simulink model "pull_rod"  (R2019b)
settings: Solver=VariableStepAuto  StartTime=0.0  StopTime=60  RelTol=1e-3
values from neighbouring files (symbols this model uses):
  b = 2000    [Aarm_Disp.m]    (also in Car_Parameters.m; PRdyn.m = 700)
  b_base = wheelbase - a    (= 0.7624)    [Aarm_Disp.m]
  bb = 2000    [Aarm_Disp.m]
  cg_height = .3987    (= 0.3987)    [Aarm_Disp.m]
  gravity = 9.81    [Aarm_Disp.m]
  H = cg_height - e    [Aarm_Disp.m]
  Kf = sf^2*ks/1375    (= 7.06492814545)    [Aarm_Disp.m]
  Kr = sr^2*ksb/1375    (= 8.08978829446)    [Aarm_Disp.m]
  ks = 52538    [Aarm_Disp.m]    (also in Car_Parameters.m = 43781.7; PRdyn.m = 43781.7)
  ksb = 61294.38    [Aarm_Disp.m]
  kt = 600    [Aarm_Disp.m]    (also in Car_Parameters.m = 81.64; PRdyn.m = 81.64)
  ktb = 600    [Aarm_Disp.m]
  l3 = .0807    (= 0.0807)    [Aarm_Disp.m]    (also in Car_Parameters.m = 0.1016; PRdyn.m = 0.1016)
  l3b = .0774    (= 0.0774)    [Aarm_Disp.m]
  l4 = .0358    (= 0.0358)    [Aarm_Disp.m]    (also in Car_Parameters.m = 0.0508; PRdyn.m = 0.0508)
  l4b = .0628    (= 0.0628)    [Aarm_Disp.m]
  mc = 63.5    [Aarm_Disp.m]    (also in Car_Parameters.m = 43; PRdyn.m = 43)
  mcb = 72.57    [Aarm_Disp.m]
  mt = 6.649    [Aarm_Disp.m]    (also in Car_Parameters.m = 12.59; PRdyn.m = 12.59)
  mtb = 11.19    [Aarm_Disp.m]
  percentage_antidive = .32    (= 0.32)    [Aarm_Disp.m]
  rch_front = 0.058    [Aarm_Disp.m]
  rch_rear = .0887    (= 0.0887)    [Aarm_Disp.m]
  total_vehicle_mass = 272.16    [Aarm_Disp.m]
  track_front = 1.168    [Aarm_Disp.m]
  track_rear = 1.143    [Aarm_Disp.m]
  wheelbase = 1.626    [Aarm_Disp.m]
undefined symbols (not defined in the file or in its folder): sigbuilder_block
settings Model: Creator=masonpesson  LastModifiedBy=masonpesson

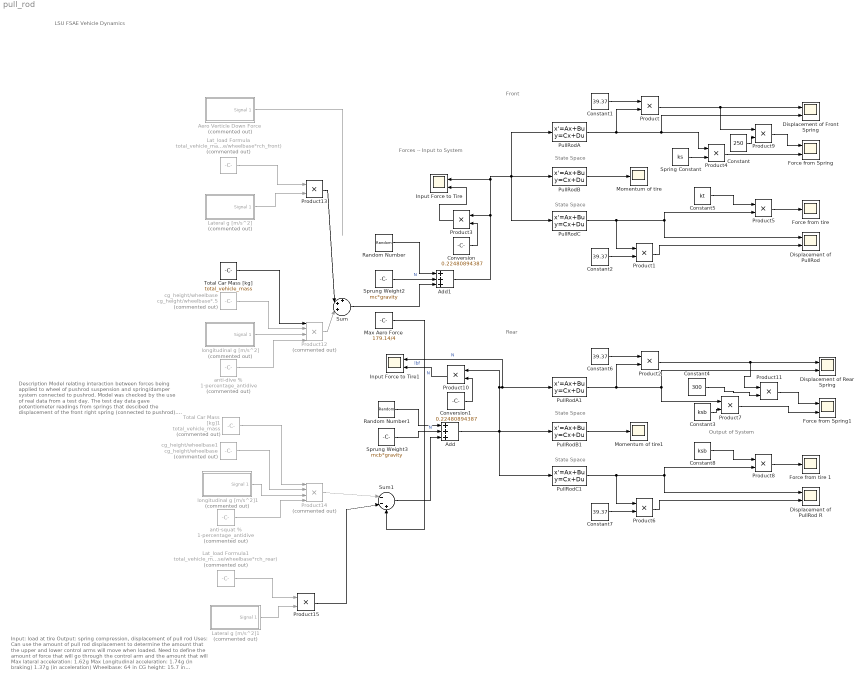
== system pull_rod ==
  note: Input: load at tire
      | Output: spring compression, displacement of pull rod
      |
      | Uses: Can use the amount of pull rod displacement to
      | determine the amount that the upper and lower control
      | arms will move when loaded.
      |
      | Need to define the amount of force that will go through
      | the control arm and the amount that will
      |
      | Max lateral acceleration: 1.62g
      | Max Longitudinal acceleration: 1.74g (in braking)
      | 								  1.37g (in acceleration)
      |
      | Wheelbase: 64 in
      | CG height: 15.7 in
      |
      | Estimated 8 % anti dive:
  note: Rear
  note: State Space
  note: Forces -- Input to System
  note: LSU FSAE Vehicle Dynamics
  note: Description
      |
      | Model relating interaction between forces being applied to wheel of pushrod suspension and spring/damper system connected to pushrod. Model was checked by the use of real data from a test day. The test day data gave potentiometer readings from springs that descibed the displacement of the front right spring (connected to pushrod). This displacement data was then used to calculate the force applied to springs. Those forces were used as an input to this model. The output the model gave was nearly identical to the actual displacment of the springs from the potentiometer data. Note that they were not exactly identical due to the model not having exact measurments but used guessed parameters. More accuate parameters will be pursued.
      |
      | Parameters
      |
      | mt %kg mass of tire --- inertia effects
      | mc %kg coner weight on tire --- force
      | kt %N/m spring in tire
      | ks %N/m spring in actual spring
      | b %Ns/m damping friction
      | l3 %m length to pull rod
      | l4 %m length to spring and damper
      | g %m/s^2 gravityGPS_Altitudem
      |
      | Found Under: Car_Parameters.m
  note: State Space
  note: State Space
  note: State Space
  note: Output of System
  note: Front
  Add : Sum  Inputs=+++
  Add1 : Sum  Inputs=+++
  Aero Verticle Down Force : Subsystem  Tag=STV Subsys  Commented=on  LoadFcn=sigbuilder_block('load');  StartFcn=sigbuilder_block('start');  StopFcn=sigbuilder_block('stop');  ClipboardFcn=sigbuilder_block('clipboard');  mask(Sigbuilder block){tuvar=[0:10]}
      mask help: Simulink:masks:SigbuilderBlock_MD
      mask init:
      | if ~strcmp(get_param(bdroot(gcbh),'SimulationStatus'),'stopped') tuvar = sigbuilder_block('maskInit'); end
      settings: CopyFcn=sigbuilder_block('copy');  DeleteFcn=sigbuilder_block('delete');  ModelCloseFcn=sigbuilder_block('modelClose');  PreSaveFcn=sigbuilder_block('preSave');  PauseFcn=sigbuilder_block('pause');  ContinueFcn=sigbuilder_block('continue');  NameChangeFcn=sigbuilder_block('namechange');  OpenFcn=sigbuilder_block('open',[437.6 199.2 550.4 400 ]);  CloseFcn=sigbuilder_block('close');
      mask Display: plot(0, 0, 100, 100,[2, 2, 32, 32, 2], [68, 8, 8, 68, 68],[32, 2], [38, 38], [32, 19, 2],[53, 60, 44], [32, 17, 17, 2],[16, 16, 31, 31]);txt = getActiveGroup(gcbh);text(2, 100, txt,'verticalAlignment', 'top');
  Constant : Constant  Value=250
  Constant{1..2,6..7} (4 alike) : Constant  Value=39.37
  Constant3 : Constant  Value=ksb
  Constant4 : Constant  Value=300
  Constant5 : Constant  Value=kt
  Constant8 : Constant  Value=ksb
  Conversion : Constant  Value=0.22480894387
  Conversion1 : Constant  Value=0.22480894387
  "Displacement of Front Spring " : Scope  NumInputPorts=2
  Displacement of PullRod : Scope  NumInputPorts=2
  Displacement of PullRod R : Scope  NumInputPorts=2
  Displacement of Rear Spring : Scope  NumInputPorts=2
  Force from Spring : Scope  NumInputPorts=2
  Force from Spring1 : Scope  NumInputPorts=2
  "Force from tire " : Scope
  Force from tire 1 : Scope
  Input Force to Tire : Scope  NumInputPorts=2
  Input Force to Tire1 : Scope  NumInputPorts=2
  Lat_load Formula : Constant  Commented=on  Value=total_vehicle_mass/track_front*((H*Kf/(Kf+Kr)) + b_base/wheelbase*rch_front)
  Lat_load Formula1 : Constant  Commented=on  Value=total_vehicle_mass/track_rear*((H*Kr/(Kr+Kf)) + b_base/wheelbase*rch_rear)
  Lateral g [m/s^2] : Subsystem  Tag=STV Subsys  Commented=on  LoadFcn=sigbuilder_block('load');  StartFcn=sigbuilder_block('start');  StopFcn=sigbuilder_block('stop');  ClipboardFcn=sigbuilder_block('clipboard');  mask(Sigbuilder block){tuvar=[0:10]}
      mask help: Simulink:masks:SigbuilderBlock_MD
      mask init:
      | if ~strcmp(get_param(bdroot(gcbh),'SimulationStatus'),'stopped') tuvar = sigbuilder_block('maskInit'); end
      settings: CopyFcn=sigbuilder_block('copy');  DeleteFcn=sigbuilder_block('delete');  ModelCloseFcn=sigbuilder_block('modelClose');  PreSaveFcn=sigbuilder_block('preSave');  PauseFcn=sigbuilder_block('pause');  ContinueFcn=sigbuilder_block('continue');  NameChangeFcn=sigbuilder_block('namechange');  OpenFcn=sigbuilder_block('open',[437.6 199.2 550.4 400 ]);  CloseFcn=sigbuilder_block('close');
      mask Display: plot(0, 0, 100, 100,[2, 2, 32, 32, 2], [68, 8, 8, 68, 68],[32, 2], [38, 38], [32, 19, 2],[53, 60, 44], [32, 17, 17, 2],[16, 16, 31, 31]);txt = getActiveGroup(gcbh);text(2, 100, txt,'verticalAlignment', 'top');
  Lateral g [m/s^2]1 : Subsystem  Tag=STV Subsys  Commented=on  LoadFcn=sigbuilder_block('load');  StartFcn=sigbuilder_block('start');  StopFcn=sigbuilder_block('stop');  ClipboardFcn=sigbuilder_block('clipboard');  mask(Sigbuilder block){tuvar=[0:10]}
      mask help: Simulink:masks:SigbuilderBlock_MD
      mask init:
      | if ~strcmp(get_param(bdroot(gcbh),'SimulationStatus'),'stopped') tuvar = sigbuilder_block('maskInit'); end
      settings: CopyFcn=sigbuilder_block('copy');  DeleteFcn=sigbuilder_block('delete');  ModelCloseFcn=sigbuilder_block('modelClose');  PreSaveFcn=sigbuilder_block('preSave');  PauseFcn=sigbuilder_block('pause');  ContinueFcn=sigbuilder_block('continue');  NameChangeFcn=sigbuilder_block('namechange');  OpenFcn=sigbuilder_block('open',[437.6 199.2 550.4 400 ]);  CloseFcn=sigbuilder_block('close');
      mask Display: plot(0, 0, 100, 100,[2, 2, 32, 32, 2], [68, 8, 8, 68, 68],[32, 2], [38, 38], [32, 19, 2],[53, 60, 44], [32, 17, 17, 2],[16, 16, 31, 31]);txt = getActiveGroup(gcbh);text(2, 100, txt,'verticalAlignment', 'top');
  Max Aero Force : Constant  Value=179.14/4
  Momentum of tire : Scope
  Momentum of tire1 : Scope
  Product{,1..11,13,15} (14 alike) : Product
  Product12 : Product  Commented=on  Inputs=4
  Product14 : Product  Commented=on  Inputs=4
  PullRodA : StateSpace  A=[0 l3/(l4*mt) 0; -l3/l4*ks -(l3/l4)^2*b/mt -kt; 0 1/mt 0]  B=[0; 1; 0]  C=[1 0 0]  D=0  InitialCondition=0
  PullRodA1 : StateSpace  A=[0 l3b/(l4b*mtb) 0; -l3b/l4b*ksb -(l3b/l4b)^2*bb/mtb -ktb; 0 1/mtb 0]  B=[0; 1; 0]  C=[1 0 0]  D=0  InitialCondition=0
  PullRodB : StateSpace  A=[0 l3/(l4*mt) 0; -l3/l4*ks -(l3/l4)^2*b/mt -kt; 0 1/mt 0]  B=[0; 1; 0]  C=[0 1 0]  D=0  InitialCondition=0
  PullRodB1 : StateSpace  A=[0 l3b/(l4b*mtb) 0; -l3b/l4b*ksb -(l3b/l4b)^2*bb/mtb -ktb; 0 1/mtb 0]  B=[0; 1; 0]  C=[0 1 0]  D=0  InitialCondition=0
  PullRodC : StateSpace  A=[0 l3/(l4*mt) 0; -l3/l4*ks -(l3/l4)^2*b/mt -kt; 0 1/mt 0]  B=[0; 1; 0]  C=[0 0 1]  D=0  InitialCondition=0
  PullRodC1 : StateSpace  A=[0 l3b/(l4b*mtb) 0; -l3b/l4b*ksb -(l3b/l4b)^2*bb/mtb -ktb; 0 1/mtb 0]  B=[0; 1; 0]  C=[0 0 1]  D=0  InitialCondition=0
  Random Number : RandomNumber  Variance=200  SampleTime=.7
  Random Number1 : RandomNumber  Variance=200  SampleTime=.7
  Spring Constant : Constant  Value=ks
  Sprung Weight2 : Constant  Value=mc*gravity
  Sprung Weight3 : Constant  Value=mcb*gravity
  Sum : Sum  Inputs=+++|
  Sum1 : Sum  Inputs=|--+
  Total Car Mass [kg] : Constant  Value=total_vehicle_mass
  Total Car Mass [kg]1 : Constant  Commented=on  Value=total_vehicle_mass
  anti-dive % : Constant  Commented=on  Value=1-percentage_antidive
  anti-squat % : Constant  Commented=on  Value=1-percentage_antidive
  cg_height/wheelbase : Constant  Commented=on  Value=cg_height/wheelbase*.5
  cg_height/wheelbase1 : Constant  Commented=on  Value=cg_height/wheelbase
  longitudinal g [m/s^2] : Subsystem  Tag=STV Subsys  Commented=on  LoadFcn=sigbuilder_block('load');  StartFcn=sigbuilder_block('start');  StopFcn=sigbuilder_block('stop');  ClipboardFcn=sigbuilder_block('clipboard');  mask(Sigbuilder block){tuvar=[0:10]}
      mask help: Simulink:masks:SigbuilderBlock_MD
      mask init:
      | if ~strcmp(get_param(bdroot(gcbh),'SimulationStatus'),'stopped') tuvar = sigbuilder_block('maskInit'); end
      settings: CopyFcn=sigbuilder_block('copy');  DeleteFcn=sigbuilder_block('delete');  ModelCloseFcn=sigbuilder_block('modelClose');  PreSaveFcn=sigbuilder_block('preSave');  PauseFcn=sigbuilder_block('pause');  ContinueFcn=sigbuilder_block('continue');  NameChangeFcn=sigbuilder_block('namechange');  OpenFcn=sigbuilder_block('open',[437.6 199.2 550.4 400 ]);  CloseFcn=sigbuilder_block('close');
      mask Display: plot(0, 0, 100, 100,[2, 2, 32, 32, 2], [68, 8, 8, 68, 68],[32, 2], [38, 38], [32, 19, 2],[53, 60, 44], [32, 17, 17, 2],[16, 16, 31, 31]);txt = getActiveGroup(gcbh);text(2, 100, txt,'verticalAlignment', 'top');
  longitudinal g [m/s^2]1 : Subsystem  Tag=STV Subsys  Commented=on  LoadFcn=sigbuilder_block('load');  StartFcn=sigbuilder_block('start');  StopFcn=sigbuilder_block('stop');  ClipboardFcn=sigbuilder_block('clipboard');  mask(Sigbuilder block){tuvar=[0:10]}
      mask help: Simulink:masks:SigbuilderBlock_MD
      mask init:
      | if ~strcmp(get_param(bdroot(gcbh),'SimulationStatus'),'stopped') tuvar = sigbuilder_block('maskInit'); end
      settings: CopyFcn=sigbuilder_block('copy');  DeleteFcn=sigbuilder_block('delete');  ModelCloseFcn=sigbuilder_block('modelClose');  PreSaveFcn=sigbuilder_block('preSave');  PauseFcn=sigbuilder_block('pause');  ContinueFcn=sigbuilder_block('continue');  NameChangeFcn=sigbuilder_block('namechange');  OpenFcn=sigbuilder_block('open',[437.6 199.2 550.4 400 ]);  CloseFcn=sigbuilder_block('close');
      mask Display: plot(0, 0, 100, 100,[2, 2, 32, 32, 2], [68, 8, 8, 68, 68],[32, 2], [38, 38], [32, 19, 2],[53, 60, 44], [32, 17, 17, 2],[16, 16, 31, 31]);txt = getActiveGroup(gcbh);text(2, 100, txt,'verticalAlignment', 'top');
  wires:
  PullRodA/1 -> Product/2, Product4/1, "Displacement of Front Spring "/2
  PullRodB/1 -> Momentum of tire/1
  Constant1/1 -> Product/1
  PullRodC/1 -> Product1/1, Product5/2, Displacement of PullRod/1
  Product1/1 -> Displacement of PullRod/2
  Constant2/1 -> Product1/2
  Conversion/1 -> Product3/2
  Spring Constant/1 -> Product4/2
  Product4/1 -> Force from Spring/2
  Constant5/1 -> Product5/1
  Product5/1 -> "Force from tire "/1
  Add1/1 -> PullRodB/1, PullRodA/1, PullRodC/1, Input Force to Tire/1, Product3/1
  Product2/1 -> Product11/1, Displacement of Rear Spring/1
  PullRodB1/1 -> Momentum of tire1/1
  Constant7/1 -> Product6/2
  Constant3/1 -> Product7/2
  Constant8/1 -> Product8/1
  Product6/1 -> Displacement of PullRod R/2
  Constant6/1 -> Product2/1
  PullRodC1/1 -> Product6/1, Product8/2, Displacement of PullRod R/1
  Product7/1 -> Force from Spring1/2
  Product8/1 -> Force from tire 1/1
  PullRodA1/1 -> Product2/2, Product7/1, Displacement of Rear Spring/2
  Product/1 -> Product9/1, "Displacement of Front Spring "/1
  Sprung Weight2/1 -> Add1/2  "N"
  Sprung Weight3/1 -> Add/2  "N"
  Constant/1 -> Product9/2
  Product9/1 -> Force from Spring/1
  Product3/1 -> Input Force to Tire/2
  Conversion1/1 -> Product10/2
  Add/1 -> Product10/1, Input Force to Tire1/1, PullRodA1/1, PullRodC1/1, PullRodB1/1  "N"
  Product10/1 -> Input Force to Tire1/2  "lbf"
  Constant4/1 -> Product11/2
  Product11/1 -> Force from Spring1/1
  Random Number/1 -> Add1/1
  Total Car Mass [kg]/1 -> Product12/1
  cg_height/wheelbase/1 -> Product12/2
  longitudinal g [m/s^2]/1(Signal 1) -> Product12/3
  Product12/1 -> Sum/3
  anti-dive %/1 -> Product12/4
  Lat_load Formula/1 -> Product13/1
  Lateral g [m/s^2]/1(Signal 1) -> Product13/2
  Product13/1 -> Sum/2
  Sum/1 -> Add1/3
  Aero Verticle Down Force/1(Signal 1) -> ?
  Total Car Mass [kg]1/1 -> Product14/1
  cg_height/wheelbase1/1 -> Product14/2
  longitudinal g [m/s^2]1/1(Signal 1) -> Product14/3
  anti-squat %/1 -> Product14/4
  Product14/1 -> Sum1/1
  Sum1/1 -> Add/3
  Random Number1/1 -> Add/1
  Lat_load Formula1/1 -> Product15/1
  Lateral g [m/s^2]1/1(Signal 1) -> Product15/2
  Product15/1 -> Sum1/2
  Max Aero Force/1 -> Sum1/3  "N"

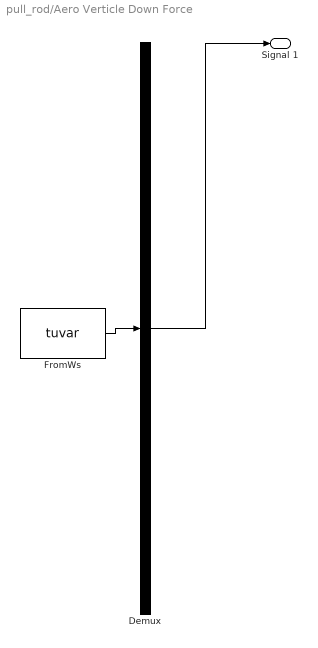
== system pull_rod/Aero Verticle Down Force ==
  Demux : Demux  Tag=STV Demux  Outputs=1
  FromWs : FromWorkspace  Tag=STV FromWs  VariableName=tuvar  SampleTime=0
      SigBuilderData=|
      | common.afterFinalStr = 'Extrapolate'
      | common.sampleTime = 0
      | dataSet.timeRange = [0 60]
      | dataSet.name = 'Group 1'
      | sbobj.Groups.Name = 'Group 1'
      | sbobj.Groups.Signals.Name = 'Signal 1'
      | sbobj.Groups.Signals.XData = [0 4 4 5 6 6 25 30 40 40 45 45 50 60]
      | sbobj.Groups.Signals.YData = [0 0 0.66 1 6 14.8 14.8 14.6 14.6 16.8 14.4 14 16 0]
      | sbobj.Groups.TimeRange = [0 60]
  Signal 1 : Outport  Tag=STV Outport
  wires:
  Demux/1 -> Signal 1/1
  FromWs/1 -> Demux/1

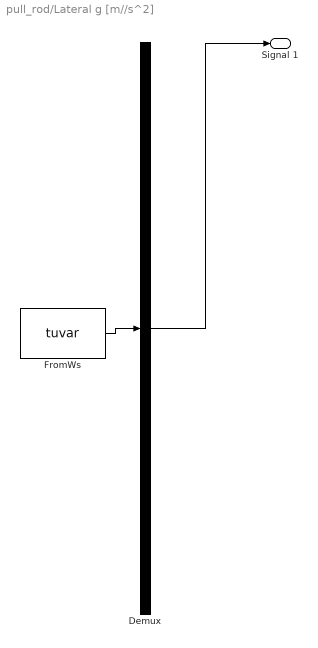
== system pull_rod/Lateral g [m//s^2] ==
  Demux : Demux  Tag=STV Demux  Outputs=1
  FromWs : FromWorkspace  Tag=STV FromWs  VariableName=tuvar  SampleTime=0
      SigBuilderData=|
      | common.afterFinalStr = 'Extrapolate'
      | common.sampleTime = 0
      | dataSet.timeRange = [0 60]
      | dataSet.name = 'Group 1'
      | sbobj.Groups.Name = 'Group 1'
      | sbobj.Groups.Signals.Name = 'Signal 1'
      | sbobj.Groups.Signals.XData = [0 4 4 5 6 6 25 30 40 40 45 45 50 60]
      | sbobj.Groups.Signals.YData = [0 0 0.66 1 6 14.8 14.8 14.6 14.6 16.8 14.4 14 16 0]
      | sbobj.Groups.TimeRange = [0 60]
  Signal 1 : Outport  Tag=STV Outport
  wires:
  Demux/1 -> Signal 1/1
  FromWs/1 -> Demux/1

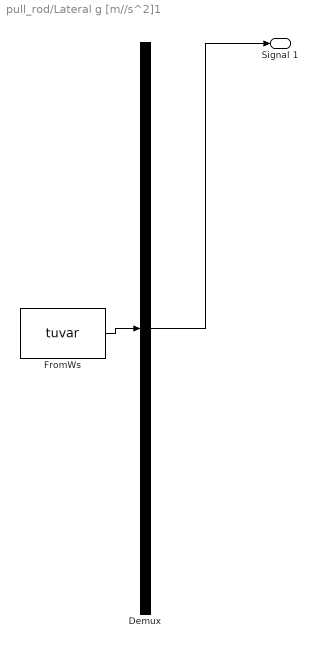
== system pull_rod/Lateral g [m//s^2]1 ==
  Demux : Demux  Tag=STV Demux  Outputs=1
  FromWs : FromWorkspace  Tag=STV FromWs  VariableName=tuvar  SampleTime=0
      SigBuilderData=|
      | common.afterFinalStr = 'Extrapolate'
      | common.sampleTime = 0
      | dataSet.timeRange = [0 60]
      | dataSet.name = 'Group 1'
      | sbobj.Groups.Name = 'Group 1'
      | sbobj.Groups.Signals.Name = 'Signal 1'
      | sbobj.Groups.Signals.XData = [0 4 4 5 6 25 25 30 40 40 45 45 50 60]
      | sbobj.Groups.Signals.YData = [0 0 0.66 1 5.25 5.4 4.2 4.4 4.2 4.4 4.4 4.6 4 0]
      | sbobj.Groups.TimeRange = [0 60]
  Signal 1 : Outport  Tag=STV Outport
  wires:
  Demux/1 -> Signal 1/1
  FromWs/1 -> Demux/1

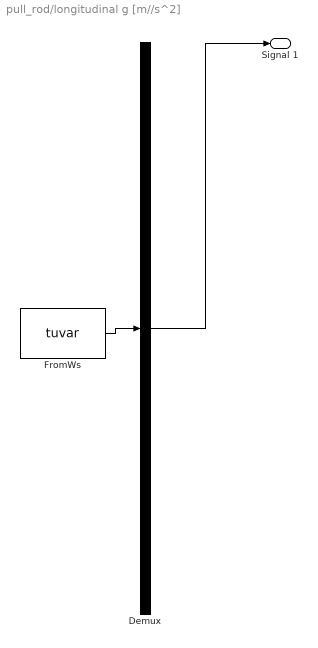
== system pull_rod/longitudinal g [m//s^2] ==
  Demux : Demux  Tag=STV Demux  Outputs=1
  FromWs : FromWorkspace  Tag=STV FromWs  VariableName=tuvar  SampleTime=0
      SigBuilderData=|
      | common.afterFinalStr = 'Extrapolate'
      | common.sampleTime = 0
      | dataSet.timeRange = [0 60]
      | dataSet.name = 'Group 1'
      | sbobj.Groups.Name = 'Group 1'
      | sbobj.Groups.Signals.Name = 'Signal 1'
      | sbobj.Groups.Signals.XData = [0 4 4 5 6 6 25 30 40 40 45 45 50 60]
      | sbobj.Groups.Signals.YData = [0 0 0.66 1 6 14.8 14.8 14.6 14.6 16.8 14.4 14 16 0]
      | sbobj.Groups.TimeRange = [0 60]
  Signal 1 : Outport  Tag=STV Outport
  wires:
  Demux/1 -> Signal 1/1
  FromWs/1 -> Demux/1

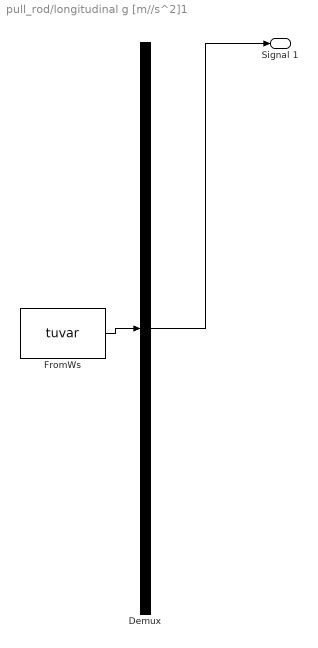
== system pull_rod/longitudinal g [m//s^2]1 ==
  Demux : Demux  Tag=STV Demux  Outputs=1
  FromWs : FromWorkspace  Tag=STV FromWs  VariableName=tuvar  SampleTime=0
      SigBuilderData=|
      | common.afterFinalStr = 'Extrapolate'
      | common.sampleTime = 0
      | dataSet.timeRange = [0 60]
      | dataSet.name = 'Group 1'
      | sbobj.Groups.Name = 'Group 1'
      | sbobj.Groups.Signals.Name = 'Signal 1'
      | sbobj.Groups.Signals.XData = [0 4 4 5 6 6 25 25 30 30 40 40 45 50 50 60]
      | sbobj.Groups.Signals.YData = [0 0 0.66 1 6 10.8 11.1 11.3 11.6 11.4 11.5 11.8 11.9 12.2 12 11.9]
      | sbobj.Groups.TimeRange = [0 60]
  Signal 1 : Outport  Tag=STV Outport
  wires:
  Demux/1 -> Signal 1/1
  FromWs/1 -> Demux/1
